simulink model "straight_forward_uniform_wind"  (R2020b)
settings: Solver=VariableStepAuto  StartTime=0.0  StopTime=10.0  RelTol=1e-3
settings Model: Creator=Dogukan  LastModifiedBy=Dogukan

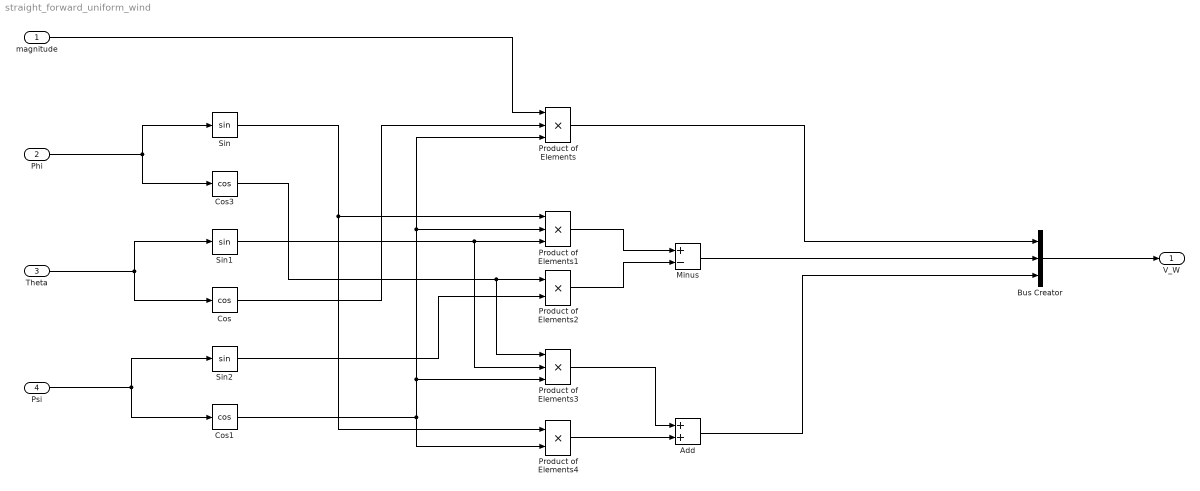
== system straight_forward_uniform_wind ==
  magnitude : Inport
  Phi : Inport  Port=2
  Theta : Inport  Port=3
  Psi : Inport  Port=4
  Add : Sum
  Bus Creator : BusCreator  Inputs=3
  Cos : Trigonometry  Operator=cos
  Cos1 : Trigonometry  Operator=cos
  Cos3 : Trigonometry  Operator=cos
  Minus : Sum  Inputs=+-
  Product of Elements : Product  Inputs=***
  Product of Elements1 : Product  Inputs=***
  Product of Elements2 : Product  Inputs=**
  Product of Elements3 : Product  Inputs=***
  Product of Elements4 : Product  Inputs=**
  Sin : Trigonometry
  Sin1 : Trigonometry
  Sin2 : Trigonometry
  V_W : Outport
  wires:
  Bus Creator/1 -> V_W/1
  Theta/1 -> Cos/1, Sin1/1
  Phi/1 -> Cos3/1, Sin/1
  Psi/1 -> Sin2/1, Cos1/1
  magnitude/1 -> Product of Elements/1
  Cos/1 -> Product of Elements/2
  Cos1/1 -> Product of Elements4/2, Product of Elements1/2, Product of Elements/3, Product of Elements3/3
  Product of Elements/1 -> Bus Creator/1
  Sin/1 -> Product of Elements4/1, Product of Elements1/1
  Sin1/1 -> Product of Elements3/2, Product of Elements1/3
  Product of Elements1/1 -> Minus/1
  Product of Elements2/1 -> Minus/2
  Product of Elements3/1 -> Add/1
  Product of Elements4/1 -> Add/2
  Minus/1 -> Bus Creator/2
  Add/1 -> Bus Creator/3
  Cos3/1 -> Product of Elements3/1, Product of Elements2/1
  Sin2/1 -> Product of Elements2/2
